simulink model "eg_9_05_R2023a"  (R2023a)
settings: Solver=ode4  StartTime=0.0  StopTime=4  FixedStep=0.001  RelTol=1e-3  EnableMultiTasking=on
values from neighbouring files (symbols this model uses):
  A = [   0  1 ... (first row only)    [eg_9_01.m]    (also in eg_9_02.m = [     0      1; eg_9_03.m = [     0      1; eg_9_04.m = [     0      1; eg_9_05.m = [     0      1)
  B = [  0 ... (first row only)    [eg_9_02.m]    (also in eg_9_03.m; eg_9_04.m; eg_9_05.m)
  K_LQ = - inv(R)*B'*P    [eg_9_04.m]    (also in eg_9_05.m = - lqr(A,B,Q,R))
  K_opt = F_opt*inv(X_opt)    [eg_9_04.m]    (also in eg_9_05.m)
  x0 = [ 1 ... (first row only)    [eg_9_05.m]
settings Model: Creator=kawata  LastModifiedBy=kawata
settings SolverCC: AlgebraicLoopSolver=TrustRegion
settings DataIOCC: SaveFormat=Array  SignalLoggingSaveFormat=ModelDataLogs  ReturnWorkspaceOutputs=off  SignalLoggingName=sigsOut
settings OptimizationCC: ExpressionDepthLimit=2147483647  LifeSpan=inf
settings DebuggingCC: SaveWithParameterizedLinksMsg=none  UnderspecifiedInitializationDetection=Classic  MergeDetectMultiDrivingBlocksExec=none  SignalResolutionControl=TryResolveAllWithWarning  MultiTaskDSMMsg=warning  MultiTaskCondExecSysMsg=none  FcnCallInpInsideContextMsg=warning  UnconnectedInputMsg=warning  UnconnectedOutputMsg=warning  UnconnectedLineMsg=warning  StateNameClashWarn=warning  SFUnexpectedBacktrackingDiag=warning  SFNoUnconditionalDefaultTransitionDiag=warning  SFExecutionAtInitializationDiag=none  ArithmeticOperatorsInVariantConditions=warning
settings HardwareCC: ProdBitPerPointer=32  ProdBitPerSizeT=32  ProdBitPerPtrDiffT=32  ProdLargestAtomicFloat=None  ProdIntDivRoundTo=Undefined  ProdEndianess=Unspecified  ProdWordSize=32  ProdHWDeviceType=32-bit Generic  TargetUnknown=on
settings ModelReferenceCC: EnableRefExpFcnMdlSchedulingChecks=on  PropagateSignalLabelsOutOfModel=off
settings SFSimCC: SimUseLocalCustomCode=off  CustomCodeUndefinedFunction=UseInterfaceOnly
settings RTWCC: RTWUseLocalCustomCode=off
settings CodeAppCC: StateflowObjectComments=on
settings GRTTargetCC: TargetLangStandard=C89/C90 (ANSI)  CombineOutputUpdateFcns=off  GRTInterface=on
settings ConfigComp: CovMetricSettings=dw  CovSaveCumulativeToWorkspaceVar=on  CovSaveSingleToWorkspaceVar=on  CovExternalEMLEnable=off

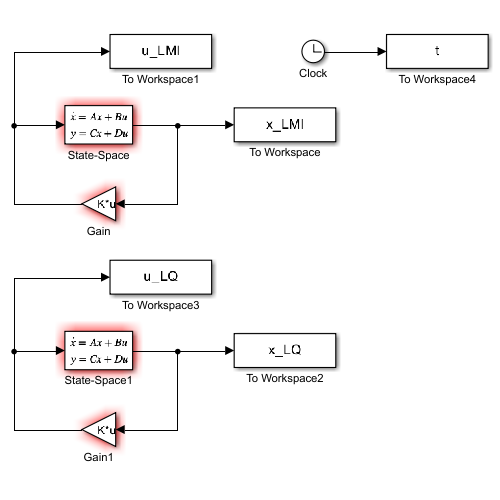
[thumbnail: Simulink's stored preview of the top-level diagram]
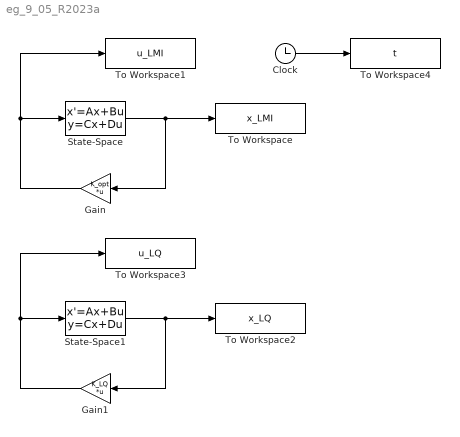
== system eg_9_05_R2023a ==
  Clock : Clock
  Gain : Gain  Gain=K_opt  Multiplication=Matrix(K*u)  SaturateOnIntegerOverflow=on  OutDataTypeStr=Inherit: Same as input  ParamDataTypeStr=Inherit: Same as input
  Gain1 : Gain  Gain=K_LQ  Multiplication=Matrix(K*u)  SaturateOnIntegerOverflow=on  OutDataTypeStr=Inherit: Same as input  ParamDataTypeStr=Inherit: Same as input
  State-Space : StateSpace  A=A  B=B  C=eye(2)  D=zeros(2,1)  InitialCondition=x0
  State-Space1 : StateSpace  A=A  B=B  C=eye(2)  D=zeros(2,1)  InitialCondition=x0
  To Workspace : ToWorkspace  VariableName=x_LMI  SampleTime=-1
  To Workspace1 : ToWorkspace  VariableName=u_LMI  SampleTime=-1
  To Workspace2 : ToWorkspace  VariableName=x_LQ  SampleTime=-1
  To Workspace3 : ToWorkspace  VariableName=u_LQ  SampleTime=-1
  To Workspace4 : ToWorkspace  VariableName=t  SampleTime=-1
  wires:
  State-Space/1 -> To Workspace/1, Gain/1
  Gain/1 -> To Workspace1/1, State-Space/1
  State-Space1/1 -> To Workspace2/1, Gain1/1
  Gain1/1 -> To Workspace3/1, State-Space1/1
  Clock/1 -> To Workspace4/1
